simulink model "CAL_3a"  (R2023a)
settings: Solver=ode4  StartTime=0.0  StopTime=105  FixedStep=0.005  RelTol=1e-3
InitFcn:
  | CAL3
values from neighbouring files (symbols this model uses):
  K_scheduled = zeros(length(V_op), 2)    [CAL3.m]    (also in CUB.m; DLC2.m; MUS.m; OHZ.m)
  kappa_track = [zeros(200,1); ones(length(theta_circ)-1, 1)/R_track]    [CAL3.m]    (also in DLC2.m = movmean(kappa_raw, 50); MUS.m = [0; 0]; OHZ.m = [0; 0]; RMP.m = [0; 0])
  psi_track = [zeros(200,1); theta_circ(2:end) + pi/2]    [CAL3.m]    (also in MUS.m = [0; 0]; OHZ.m = [0; 0]; RMP.m = [0; 0]; SLA.m = atan2(dy_ds, dx_ds))
  s_track = [0; cumsum(sqrt(dx.^2 + dy.^2))]    [CAL3.m]    (also in MUS.m = [0; 2000]; OHZ.m = [0; 2000]; RMP.m = [0; 2000]; SLA.m)
  V_op = 5:5:85    [CAL3.m]    (also in CUB.m; DLC2.m; MUS.m; OHZ.m)
  V_profile = conv(V_profile, ones(window_size,1)/window_size, 'same')    [CAL3.m]    (also in SLA.m = u_ms * ones(size(s_track)))
  X_track = [linspace(0, runway_length, 200)'; runway_length + R_track * cos(theta_circ(2:end))]    [CAL3.m]    (also in CUB.m = [0; 5000]; DLC2.m = 0:0.1:total_track_length; MUS.m = [0; 2000]; OHZ.m = [0; 2000])
  Y_track = [zeros(200, 1); R_track + R_track * sin(theta_circ(2:end))]    [CAL3.m]    (also in CUB.m = [0; 0]; DLC2.m = zeros(size(X_track)); MUS.m = [0; 0]; OHZ.m = [0; 0])
undefined symbols (not defined in the file or in its folder): veh_params
libraries: simulink x2, slpidlib x1
(part 2 of 2)

== matlab function CAL_3a/Scopes/MATLAB Function1 ==
  settings: updateMethod=DISCRETE
  data: delta input; psi input; psi_ref input; Fx input; Fy input; Fz input; Trl input; Trr input; Tf_f input; Trl_f input; Trr_f input; w_vec input; vx input; vy input; ax input; ay input
function vehicle_frame_plotter(delta, psi, psi_ref, Fx, Fy, Fz, Trl, Trr, Tf_f, Trl_f, Trr_f, w_vec, vx, vy, ax, ay)
    coder.extrinsic('figure', 'plot', 'hold', 'axis', 'title', 'set', 'drawnow', 'patch', 'text', 'line', 'quiver', 'sprintf');
    
    persistent hWheels hSteer hSpokes hPsiRef hPsiAct hFlags hTqFlags hMotors hAxleFront hCircles hGdots hSwLabel hRwLabel hAngleLabel hVelArrow hAccArrow hVelText hAccText hCrosshairs counter
    
    if isempty(counter)
        % =====================================================================
        % STRICT CODER INITIALIZATION
        % =====================================================================
        counter = 0;
        hSteer = 0.0; hPsiRef = 0.0; hPsiAct = 0.0; hAxleFront = 0.0;
        hWheels = zeros(1,4); hFlags = zeros(1,4); hTqFlags = zeros(1,2); hMotors = zeros(1,2);
        hSpokes = zeros(1,3); hCircles = zeros(1,4); hGdots = zeros(1,4);
        hSwLabel = 0.0; hRwLabel = 0.0; hAngleLabel = 0.0;
        hVelArrow = 0.0; hAccArrow = 0.0; hVelText = 0.0; hAccText = 0.0;
        hCrosshairs = zeros(1,2);
        
        figure('Name', 'Vehicle Frame Telemetry - Car A', 'Color', 'w', 'Position', [100, 100, 750, 750]);
        hold on;
        
        % Chassis Outline & Front Axle
        plot([-1, 1, 1, -1, -1], [2, 2, -2, -2, 2], 'k', 'LineWidth', 2);
        hAxleFront = double(line([1, -1], [1.5, 1.5], 'Color', [0.2 0.2 0.2], 'LineWidth', 2));
        
        % Wheels Array Setup [FL, FR, RL, RR]
        for i = 1:4; hWheels(i) = double(patch(0, 0, [0.3 0.3 0.3])); end
        
        % =====================================================================
        % FRICTION CIRCLES, STEERING WHEEL, & YAW VECTORS
        % =====================================================================
        th_c = 0:0.1:2*pi;
        circle_x = cos(th_c); circle_y = sin(th_c);
        c_pos = [-2.0, 2.3; 2.0, 2.3; -2.0, -2.3; 2.0, -2.3]; 
        for i = 1:4
            hCircles(i) = double(plot(c_pos(i,1) + 0.5*circle_x, c_pos(i,2) + 0.5*circle_y, 'Color', [0.6 0 0.6], 'LineStyle', '--', 'LineWidth', 1.2));
            hGdots(i) = double(plot(c_pos(i,1), c_pos(i,2), 'mo', 'MarkerFaceColor', 'm', 'MarkerSize', 5));
        end
        
        hSteer = double(plot(0.4*cos(th_c), 0.4*sin(th_c) + 0.5, 'k', 'LineWidth', 3));
        hSpokes(1) = double(line([0, 0], [0.5, 0.5], 'Color', 'k', 'LineWidth', 2.5));
        hSpokes(2) = double(line([0, 0], [0.5, 0.5], 'Color', 'k', 'LineWidth', 2.5));
        hSpokes(3) = double(line([0, 0], [0.5, 0.5], 'Color', 'k', 'LineWidth', 2.5));
        
        hPsiRef = double(quiver(0, 1.8, 0, 0.8, 'r', 'LineWidth', 2.5, 'MaxHeadSize', 2));
        hPsiAct = double(quiver(0, 1.8, 0, 0.8, 'b', 'LineWidth', 2.5, 'MaxHeadSize', 2));
        
        for i = 1:4; hFlags(i) = double(text(0, 0, '', 'FontSize', 8, 'BackgroundColor', [1 1 1 0.8], 'EdgeColor', 'k')); end
        
        % =====================================================================
        % VEHICLE A POWERTRAIN GRAPHIC (Dual Motors)
        % =====================================================================
        m_b = [-.15, .15, .15, -.15]; m_w = [.2, .2, -.2, -.2];
        hMotors(1) = double(patch(m_b - 0.6, m_w - 1.5, [0.5 0.5 0.5])); % Left Motor
        hMotors(2) = double(patch(m_b + 0.6, m_w - 1.5, [0.5 0.5 0.5])); % Right Motor
        
        hTqFlags(1) = double(text(-0.6, -0.9, '', 'FontSize', 10, 'FontWeight', 'bold', 'HorizontalAlignment', 'center'));
        hTqFlags(2) = double(text(0.6, -0.9, '', 'FontSize', 10, 'FontWeight', 'bold', 'HorizontalAlignment', 'center'));
        
        % Labels
        hSwLabel = double(text(0, 1.2, '', 'FontSize', 9, 'FontWeight', 'bold', 'HorizontalAlignment', 'center'));
        hRwLabel = double(text(0, 1.65, '', 'FontSize', 9, 'FontWeight', 'bold', 'HorizontalAlignment', 'center', 'Color', [0 0.5 0]));
        hAngleLabel = double(text(0, 2.8, '', 'FontSize', 10, 'FontWeight', 'bold', 'HorizontalAlignment', 'center', 'Color', [0.4 0 0.6]));

        % =====================================================================
        % SHARED-ORIGIN VELOCITY & ACCELERATION VECTORS
        % =====================================================================
        hCrosshairs(1) = double(plot([-2.0 2.0], [-3.8 -3.8], 'k:', 'Color', [0.7 0.7 0.7]));
        hCrosshairs(2) = double(plot([0 0], [-4.2 -1.8], 'k:', 'Color', [0.7 0.7 0.7]));

        hVelArrow = double(quiver(0, -3.8, 0, 0, 'Color', [0 0.4 0.8], 'LineWidth', 2.5, 'MaxHeadSize', 2, 'AutoScale', 'off'));
        hAccArrow = double(quiver(0, -3.8, 0, 0, 'Color', [0.8 0.3 0], 'LineWidth', 2.5, 'MaxHeadSize', 2, 'AutoScale', 'off'));

        hVelText = double(text(-2.0, -4.3, '', 'FontSize', 9, 'FontWeight', 'bold', 'HorizontalAlignment', 'center', 'Color', [0 0.4 0.8]));
        hAccText = double(text(2.0, -4.3, '', 'FontSize', 9, 'FontWeight', 'bold', 'HorizontalAlignment', 'center', 'Color', [0.8 0.3 0]));
        
        axis([-4.5 4.5 -4.5 4.5]); axis equal; grid on;
        title('Dynamics - Car A (Dual Motor): Forces & Friction Circles');
    end
    counter = counter + 1;
    
    % --- UPDATE LOOP ---
    if mod(counter, 10) == 0
        R_delta = [cos(delta) -sin(delta); sin(delta) cos(delta)];
        w_orig = [-.2 .2 .2 -.2; .4 .4 -.4 -.4]; 
        w_rot = R_delta * w_orig;
        
        set(hWheels(1), 'XData', w_rot(1,:) - 1, 'YData', w_rot(2,:) + 1.5); 
        set(hWheels(2), 'XData', w_rot(1,:) + 1, 'YData', w_rot(2,:) + 1.5); 
        set(hWheels(3), 'XData', w_orig(1,:) - 1, 'YData', w_orig(2,:) - 1.5); 
        set(hWheels(4), 'XData', w_orig(1,:) + 1, 'YData', w_orig(2,:) - 1.5); 
        
        set(hAxleFront, 'XData', [mean(w_rot(1,:) - 1), mean(w_rot(1,:) + 1)], 'YData', [mean(w_rot(2,:) + 1.5), mean(w_rot(2,:) + 1.5)]);
        
        sw_a = delta * 14; 
        th_sw = (0:0.1:2*pi) + sw_a;
        set(hSteer, 'XData', 0.4*cos(th_sw), 'YData', 0.4*sin(th_sw) + 0.5);
        spk = [0, pi, 1.5*pi] + sw_a;
        for j=1:3; set(hSpokes(j), 'XData', [0, 0.4*cos(spk(j))], 'YData', [0.5, 0.5 + 0.4*sin(spk(j))]); end
        
        set(hSwLabel, 'String', sprintf('SW: %.1f deg', sw_a * 180/pi));
        set(hRwLabel, 'String', sprintf('RW: %.1f deg', delta * 180/pi));
        
        psi_e = psi_ref - psi; 
        set(hPsiRef, 'UData', 0.8*sin(psi_e), 'VData', 0.8*cos(psi_e));
        set(hPsiAct, 'UData', 0, 'VData', 0.8);
        set(hAngleLabel, 'String', sprintf('Sideslip: %.1f deg', psi_e * 180/pi));
        
        fb = [abs(Tf_f/2), abs(Tf_f/2), abs(Trl_f), abs(Trr_f)]; 
        mu = 1.0;
        c_pos = [-2.0, 2.3; 2.0, 2.3; -2.0, -2.3; 2.0, -2.3]; 
        th_c = 0:0.1:2*pi;
        rpm_vec = w_vec * (30 / pi);
        
        for i = 1:4
            if fb(i) > 5; set(hWheels(i), 'FaceColor', [0.8 0 0]); else set(hWheels(i), 'FaceColor', [0.3 0.3 0.3]); end
            F_max = max(100, mu * Fz(i));
            scale = 0.5 / 6000; 
            set(hCircles(i), 'XData', c_pos(i,1) + F_max*scale*cos(th_c), 'YData', c_pos(i,2) + F_max*scale*sin(th_c));
            set(hGdots(i), 'XData', c_pos(i,1) + Fy(i)*scale, 'YData', c_pos(i,2) + Fx(i)*scale);
        end
        
        % Dual Motor Visualization Logic
        mt = [Trl, Trr]; 
        for k = 1:2
            if mt(k) > 0.1; set(hMotors(k), 'FaceColor', [0 0.7 0]); 
            elseif mt(k) < -0.1; set(hMotors(k), 'FaceColor', [0.7 0 0]); 
            else set(hMotors(k), 'FaceColor', [0.5 0.5 0.5]); end
            
            set(hTqFlags(k), 'String', sprintf('%.1f Nm', mt(k)));
        end
        
        pos = [-4.1, 1.5; 2.8, 1.5; -4.1, -1.5; 2.8, -1.5]; 
        for i = 1:4
            f_str = sprintf('Fx: %.0f\nFy: %.0f\nFz: %.0f\nFric: %.1f\nRPM: %.0f', Fx(i), Fy(i), Fz(i), fb(i), rpm_vec(i));
            set(hFlags(i), 'Position', [pos(i,1), pos(i,2)], 'String', f_str);
        end

        % =====================================================================
        % UPDATE DYNAMIC VECTORS
        % =====================================================================
        vx_kmh = vx * 3.6;
        vy_kmh = vy * 3.6;
        ax_g = ax / 9.81;
        ay_g = ay / 9.81;

        vel_scale = 0.015; 
        acc_scale = 0.8;   

        set(hVelArrow, 'UData', -vy_kmh * vel_scale, 'VData', vx_kmh * vel_scale);
        set(hAccArrow, 'UData', -ay_g * acc_scale, 'VData', ax_g * acc_scale);

        set(hVelText, 'String', sprintf('Vx: %.1f | Vy: %.1f\n[km/h]', vx_kmh, vy_kmh));
        set(hAccText, 'String', sprintf('Ax: %.2f | Ay: %.2f\n[G]', ax_g, ay_g));
        
        drawnow limitrate;
    end
end

== matlab function CAL_3a/Vehicle & Powertrain Plant1/MATLAB Function ==
  data: delta input; Trr_m input; Trl_m input; Trr_f input; Trl_f input; Tf_f input; vx input; vy input; r input; psi input; SOC input; T_batt input; T_motor input; w_fl input; w_fr input; w_rl input; w_rr input; vx_dot output; vy_dot output; r_dot output; X_dot output; Y_dot output; psi_dot output; s_dot output; SOC_dot output; T_batt_dot output; T_mot_dot output; Fz_f_tot output; Fz_r_tot output; Fz_rl output; Fz_rr output; Fx_vec output; Fy_vec output; Fz_vec output; w_vec output; w_dot_vec output; veh_params parameter; I_batt output; Pwr_Elec output
function [vx_dot, vy_dot, r_dot, X_dot, Y_dot, psi_dot, s_dot, SOC_dot, T_batt_dot, T_mot_dot, Fz_f_tot, Fz_r_tot, Fz_rl, Fz_rr, Fx_vec, Fy_vec, Fz_vec, w_vec, w_dot_vec, I_batt, Pwr_Elec] = vehicle_physics_engine(delta, Trr_m, Trl_m, Trr_f, Trl_f, Tf_f, vx, vy, r, psi, SOC, T_batt, T_motor, w_fl, w_fr, w_rl, w_rr, veh_params)
    
    % =========================================================================
    % 0. EXPLICIT OUTPUT INITIALIZATION & SCALAR COERCION 
    % =========================================================================
    vx_dot = 0.0; vy_dot = 0.0; r_dot = 0.0; 
    X_dot = 0.0; Y_dot = 0.0; psi_dot = 0.0; s_dot = 0.0;
    SOC_dot = 0.0; T_batt_dot = 0.0; T_mot_dot = 0.0;
    Fz_f_tot = 0.0; Fz_r_tot = 0.0; Fz_rl = 0.0; Fz_rr = 0.0;
    Fx_vec = zeros(1,4); Fy_vec = zeros(1,4); Fz_vec = zeros(1,4);
    w_vec = zeros(1,4); w_dot_vec = zeros(1,4);
    I_batt = 0.0; 
    Pwr_Elec = 0.0; % NEW: Output initialization for Electrical Power

    % Force scalar inputs (strips undefined array dimensions from Simulink lines)
    delta = delta(1); vx = vx(1); vy = vy(1); r = r(1); psi = psi(1);
    Trr_m = Trr_m(1); Trl_m = Trl_m(1); Trr_f = Trr_f(1); Trl_f = Trl_f(1); Tf_f = Tf_f(1);
    SOC = SOC(1); T_batt = T_batt(1); T_motor = T_motor(1);
    w_fl = w_fl(1); w_fr = w_fr(1); w_rl = w_rl(1); w_rr = w_rr(1);

    % =========================================================================
    % HIGH-FIDELITY EV VEHICLE DYNAMICS PLANT MODEL
    % =========================================================================
    
    % ---------------------------------------------------------------------
    % 1. UNPACK CENTRALIZED PARAMETERS
    % ---------------------------------------------------------------------
    m = veh_params.m(1); Iz = veh_params.Iz(1); lf = veh_params.lf(1); lr = veh_params.lr(1); L = veh_params.L(1);
    tw = veh_params.tw(1); h_cg = veh_params.h_cg(1); Rw = veh_params.Rw(1); Iw = veh_params.Iw(1); 
    G = veh_params.G(1); g = veh_params.g(1); rho = veh_params.rho(1); CdA = veh_params.CdA(1);
    roll_bias_f = veh_params.roll_bias_f(1); 
    
    mu_max = veh_params.mu_max(1); C_rr = veh_params.C_rr(1);
    ks_f = veh_params.ks_f(1)/2; ks_r = veh_params.ks_r(1)/2;
    C_tire = veh_params.C_tire(1); E_tire = veh_params.E_tire(1);
    
    if abs(vx) < 0.5
        vx_safe = 0.5 * sign(vx + 1e-6); 
    else
        vx_safe = vx;
    end
    
    F_aero_drag = 0.5 * rho * CdA * vx_safe * abs(vx_safe);
    
    % ---------------------------------------------------------------------
    % 2. DYNAMIC TIRE PEAK CALIBRATION
    % ---------------------------------------------------------------------
    Fz_axle_f_static = m * g * (lr / L); 
    Fz_axle_r_static = m * g * (lf / L); 
    
    D_tire_f = mu_max * (Fz_axle_f_static / 2); 
    D_tire_r = mu_max * (Fz_axle_r_static / 2); 
    
    B_tire_f = ks_f / (C_tire * D_tire_f * 2); 
    B_tire_r = ks_r / (C_tire * D_tire_r * 2); 
    
    % ---------------------------------------------------------------------
    % 3. 3D WEIGHT TRANSFER 
    % ---------------------------------------------------------------------
    Trr_tot = Trr_m * G + Trr_f;
    Trl_tot = Trl_m * G + Trl_f;
    Tf_tot_half = Tf_f / 2; 
    
    Fx_fl_tq = Tf_tot_half / Rw; Fx_fr_tq = Tf_tot_half / Rw;
    Fx_rl_tq = Trl_tot / Rw; Fx_rr_tq = Trr_tot / Rw;
    
    ax_est = ((Fx_fl_tq + Fx_fr_tq + Fx_rl_tq + Fx_rr_tq) - F_aero_drag) / m;
    ay_est = vx_safe * r;
    
    Fz_f_tot = m * g * (lr / L) - m * ax_est * (h_cg / L);
    Fz_r_tot = m * g * (lf / L) + m * ax_est * (h_cg / L);
    
    dFz_y_f = m * ay_est * (h_cg / tw) * roll_bias_f;
    dFz_y_r = m * ay_est * (h_cg / tw) * (1 - roll_bias_f);
    
    Fz_max_f = Fz_axle_f_static * 2.5; 
    Fz_max_r = Fz_axle_r_static * 2.5;
    
    Fz_fl = max(100, min(Fz_max_f, Fz_f_tot / 2 - dFz_y_f));
    Fz_fr = max(100, min(Fz_max_f, Fz_f_tot / 2 + dFz_y_f));
    Fz_rl = max(100, min(Fz_max_r, Fz_r_tot / 2 - dFz_y_r));
    Fz_rr = max(100, min(Fz_max_r, Fz_r_tot / 2 + dFz_y_r));
    Fz_vec = [Fz_fl, Fz_fr, Fz_rl, Fz_rr];
    
    % ---------------------------------------------------------------------
    % 4. VECTOR-SUM PACEJKA COMBINED SLIP MODEL
    % ---------------------------------------------------------------------
    v_hub_fl = vx_safe - (tw / 2) * r; v_hub_fr = vx_safe + (tw / 2) * r;
    v_hub_rl = vx_safe - (tw / 2) * r; v_hub_rr = vx_safe + (tw / 2) * r;
    
    k_fl = (w_fl * Rw - v_hub_fl) / max(abs(v_hub_fl), 1.0);
    k_fr = (w_fr * Rw - v_hub_fr) / max(abs(v_hub_fr), 1.0);
    k_rl = (w_rl * Rw - v_hub_rl) / max(abs(v_hub_rl), 1.0);
    k_rr = (w_rr * Rw - v_hub_rr) / max(abs(v_hub_rr), 1.0);
    
    alpha_fl = delta - atan((vy + lf * r) / max(abs(v_hub_fl), 1.0));
    alpha_fr = delta - atan((vy + lf * r) / max(abs(v_hub_fr), 1.0));
    alpha_rl = -atan((vy - lr * r) / max(abs(v_hub_rl), 1.0));
    alpha_rr = -atan((vy - lr * r) / max(abs(v_hub_rr), 1.0));
    
    sigma_fl = sqrt(k_fl^2 + tan(alpha_fl)^2) + 1e-6;
    sigma_fr = sqrt(k_fr^2 + tan(alpha_fr)^2) + 1e-6;
    sigma_rl = sqrt(k_rl^2 + tan(alpha_rl)^2) + 1e-6;
    sigma_rr = sqrt(k_rr^2 + tan(alpha_rr)^2) + 1e-6;
    
    F_tot_fl = mu_max * Fz_fl * sin(C_tire * atan(B_tire_f * sigma_fl - E_tire * (B_tire_f * sigma_fl - atan(B_tire_f * sigma_fl))));
    F_tot_fr = mu_max * Fz_fr * sin(C_tire * atan(B_tire_f * sigma_fr - E_tire * (B_tire_f * sigma_fr - atan(B_tire_f * sigma_fr))));
    F_tot_rl = mu_max * Fz_rl * sin(C_tire * atan(B_tire_r * sigma_rl - E_tire * (B_tire_r * sigma_rl - atan(B_tire_r * sigma_rl))));
    F_tot_rr = mu_max * Fz_rr * sin(C_tire * atan(B_tire_r * sigma_rr - E_tire * (B_tire_r * sigma_rr - atan(B_tire_r * sigma_rr))));
    
    Fx_fl = F_tot_fl * (k_fl / sigma_fl) - C_rr * Fz_fl * tanh(v_hub_fl * 10);
    Fx_fr = F_tot_fr * (k_fr / sigma_fr) - C_rr * Fz_fr * tanh(v_hub_fr * 10);
    Fx_rl = F_tot_rl * (k_rl / sigma_rl) - C_rr * Fz_rl * tanh(v_hub_rl * 10);
    Fx_rr = F_tot_rr * (k_rr / sigma_rr) - C_rr * Fz_rr * tanh(v_hub_rr * 10);
    Fx_vec = [Fx_fl, Fx_fr, Fx_rl, Fx_rr];
    
    Fy_fl = F_tot_fl * (tan(alpha_fl) / sigma_fl);
    Fy_fr = F_tot_fr * (tan(alpha_fr) / sigma_fr);
    Fy_rl = F_tot_rl * (tan(alpha_rl) / sigma_rl);
    Fy_rr = F_tot_rr * (tan(alpha_rr) / sigma_rr);
    Fy_vec = [Fy_fl, Fy_fr, Fy_rl, Fy_rr];
    
    % ---------------------------------------------------------------------
    % 5. CHASSIS & WHEEL INTEGRATORS
    % ---------------------------------------------------------------------
    w_fl_dot = (-abs(Tf_f / 2) * sign(w_fl) - Fx_fl * Rw) / Iw;
    w_fr_dot = (-abs(Tf_f / 2) * sign(w_fr) - Fx_fr * Rw) / Iw;
    w_rl_dot = (Trl_m * G - abs(Trl_f) * sign(w_rl) - Fx_rl * Rw) / Iw;
    w_rr_dot = (Trr_m * G - abs(Trr_f) * sign(w_rr) - Fx_rr * Rw) / Iw;
    w_dot_vec = [w_fl_dot, w_fr_dot, w_rl_dot, w_rr_dot];
    w_vec = [w_fl, w_fr, w_rl, w_rr];
    
    sum_Fx = (Fx_fl + Fx_fr) * cos(delta) - (Fy_fl + Fy_fr) * sin(delta) + Fx_rl + Fx_rr;
    vx_dot = (sum_Fx - F_aero_drag) / m + vy * r;
    
    sum_Fy = (Fy_fl + Fy_fr) * cos(delta) + (Fx_fl + Fx_fr) * sin(delta) + Fy_rl + Fy_rr;
    vy_dot = sum_Fy / m - vx_safe * r;
    
    M_front = lf * ((Fy_fl + Fy_fr) * cos(delta) + (Fx_fl + Fx_fr) * sin(delta));
    M_rear  = -lr * (Fy_rl + Fy_rr);
    M_tv    = (Fx_rr - Fx_rl) * (tw / 2); 
    r_dot  = (M_front + M_rear + M_tv) / Iz;
    
    X_dot   = vx_safe * cos(psi) - vy * sin(psi);
    Y_dot   = vx_safe * sin(psi) + vy * cos(psi);
    psi_dot = r;
    s_dot   = vx_safe;
    
    % ---------------------------------------------------------------------
    % 6. THERMALS & SOC (R-INT BATTERY MODEL)
    % ---------------------------------------------------------------------
    P_mech = (Trr_m + Trl_m) * G * (vx_safe / Rw);
    P_elec = P_mech; 
    
    if P_mech > 500
        P_elec = P_mech / 0.90; 
    elseif P_mech < -500
        P_elec = P_mech * 0.90; 
    end
    
    V_oc = veh_params.V_pack; 
    R_int = 0.015;            
    
    discriminant = V_oc^2 - 4 * R_int * P_elec;
    
    if discriminant < 0
        discriminant = 0;
    end
    
    I_curr = (V_oc - sqrt(discriminant)) / (2 * R_int);
    
    % NEW OUTPUTS
    I_batt = I_curr;
    Pwr_Elec = P_elec;
    
    SOC_dot = -I_curr / (veh_params.Cap_Ah * 3600);
    
    T_batt_dot = ((I_curr^2) * R_int - veh_params.hA_cool_batt * (T_batt - veh_params.T_coolant_batt)) / (veh_params.m_batt * veh_params.cp_batt);
    T_mot_dot  = (abs(P_elec - P_mech) - veh_params.hA_cool_motor * (T_motor - veh_params.T_ambient)) / (veh_params.m_motor * veh_params.cp_motor);
end

== matlab function CAL_3a/Vehicle Control Unit (VCU)/MATLAB Function ==
  settings: updateMethod=DISCRETE
  data: delta_curr input; pedal input; T_rr_motor_raw output; vx_curr input; vy_curr input; r_curr input; kappa_ref input; Fz_f_total input; Fz_r_total input; Fz_rl input; Fz_rr input; SOC input; T_batt input; T_motor input; V_op parameter; K_scheduled parameter; T_rl_motor_raw output; T_rr_fric output; w_vec input; T_rl_fric output; T_f_fric output; Mz_cmd output; r_ref output
function [T_rr_motor_raw, T_rl_motor_raw, T_rr_fric, T_rl_fric, T_f_fric, Mz_cmd, r_ref] = vcu_allocator(delta_curr, pedal, vx_curr, vy_curr, r_curr, kappa_ref, Fz_f_total, Fz_r_total, Fz_rl, Fz_rr, SOC, T_batt, T_motor, V_op, K_scheduled, w_vec)
T_rr_motor_raw = 0.0;
T_rl_motor_raw = 0.0;
T_rr_fric = 0.0;
T_rl_fric = 0.0;
T_f_fric = 0.0;
Mz_cmd = 0.0;

Rw = 0.34; tw = 1.65; G = 10; mu_max = 1.2;

% --- Per-Motor Limits (Total System = 500 kW, 800 Nm) ---
P_motor_base = 250000; % 250 kW per motor
T_motor_max = 400;     % 400 Nm per motor
T_fric_max_per_wheel = 3500;
% --------------------------------------------------------

% --- Battery and Thermal Derating ---
T_batt_cal = [-10, 0, 15, 45, 55, 60]; P_derate_batt_cal = [0, 0.5, 1.0, 1.0, 0.2, 0];
T_motor_cal = [30, 90, 110, 130, 150]; P_derate_motor_cal = [1.0, 1.0, 0.8, 0.2, 0];
SOC_vec = [0, 0.05, 0.15, 0.85, 0.95, 1.0];
P_derate_SOC_dis = [0, 0.1, 1.0, 1.0, 1.0, 1.0]; P_derate_SOC_chg = [1.0, 1.0, 1.0, 1.0, 0.1, 0];

derate_T_batt = interp1(T_batt_cal, P_derate_batt_cal, T_batt(1), 'linear', 0);
derate_T_mot = interp1(T_motor_cal, P_derate_motor_cal, T_motor(1), 'linear', 0);
derate_T_total = min(derate_T_batt, derate_T_mot);

derate_S_dis = interp1(SOC_vec, P_derate_SOC_dis, SOC(1), 'linear', 0);
derate_S_chg = interp1(SOC_vec, P_derate_SOC_chg, SOC(1), 'linear', 0);

P_avail_dis = P_motor_base * min(derate_T_total, derate_S_dis);
P_avail_chg = P_motor_base * min(derate_T_total, derate_S_chg);

vx_lqr = max(vx_curr(1), 5.0);

% --- Speed-based Torque Vectoring Blending (45 km/h to 50 km/h) ---
vx_kmh = vx_curr(1) * 3.6;
tv_blend_lower = 45.0;
tv_blend_upper = 50.0;
if vx_kmh >= tv_blend_upper
    tv_blend = 1.0;
elseif vx_kmh <= tv_blend_lower
    tv_blend = 0.0;
else
    tv_blend = (vx_kmh - tv_blend_lower) / (tv_blend_upper - tv_blend_lower);
end

% --- LQR Yaw Moment Calculation ---
K_dyn_1 = interp1(V_op, K_scheduled(:,1), vx_lqr, 'linear', 'extrap');
K_dyn_2 = interp1(V_op, K_scheduled(:,2), vx_lqr, 'linear', 'extrap');

% =========================================================================
% 1. DYNAMIC ACKERMANN REFERENCE
% =========================================================================
L = 2.6;            % Wheelbase
K_us = 0.0015;      % Small understeer gradient (optional)
r_ref_raw = (vx_lqr * delta_curr(1)) / (L * (1 + K_us * vx_lqr^2));

% =========================================================================
% 2. PHYSICAL YAW RATE BOUNDING (The Jitter Fix)
% =========================================================================
g = 9.81;
% Calculate the absolute maximum yaw rate the tires can sustain
% based on current speed and track friction (r_max = mu * g / Vx)
% We use 0.95 as a safety margin to prevent fighting the TCS limiters.
r_max_phys = (mu_max * g * 0.95) / vx_lqr;

% Clamp the reference so the LQR never demands an impossible turn
r_ref = max(-r_max_phys, min(r_max_phys, r_ref_raw));

% =========================================================================
TV_Bite_Factor = 1;
vy_factor = 1;
Mz_req = tv_blend * -(vy_factor * K_dyn_1(1) * vy_curr(1) + TV_Bite_Factor * K_dyn_2(1) * (r_curr(1) - r_ref));

Mz_cmd = max(-2500, min(2500, Mz_req));
T_delta_wheel_raw = max(-1500, min(1500, (Mz_cmd * Rw) / tw));

% =========================================================================
% --- DYNAMIC MOTOR POWER LIMITS (Hyperbolic Torque Derating) ---
% =========================================================================
% Calculate actual motor speed from wheel speed (rad/s)
% w_vec = [w_fl, w_fr, w_rl, w_rr]
w_motor_rl = max(abs(w_vec(3) * G), 0.1); % Prevent div-by-zero at standstill
w_motor_rr = max(abs(w_vec(4) * G), 0.1);

% Power-limited torque curve: T_max = P_max / w
T_limit_rl_dis = P_avail_dis / w_motor_rl;
T_limit_rr_dis = P_avail_dis / w_motor_rr;
T_limit_rl_chg = P_avail_chg / w_motor_rl;
T_limit_rr_chg = P_avail_chg / w_motor_rr;

% Final motor bounds (Minimum of Inverter current limit and Power limit)
T_motor_lim_rl_dis = min(T_motor_max, T_limit_rl_dis);
T_motor_lim_rr_dis = min(T_motor_max, T_limit_rr_dis);
T_motor_lim_rl_chg = max(-T_motor_max, -T_limit_rl_chg);
T_motor_lim_rr_chg = max(-T_motor_max, -T_limit_rr_chg);

% =========================================================================
T_grip_lim_rl_wheel = mu_max * Fz_rl(1) * Rw * 0.90;
T_grip_lim_rr_wheel = mu_max * Fz_rr(1) * Rw * 0.90;

% Combine physical motor limits with dynamic grip limits
T_max_rl_motor = min(T_motor_lim_rl_dis, T_grip_lim_rl_wheel / G);
T_max_rr_motor = min(T_motor_lim_rr_dis, T_grip_lim_rr_wheel / G);
T_min_rl_motor = max(T_motor_lim_rl_chg, -T_grip_lim_rl_wheel / G);
T_min_rr_motor = max(T_motor_lim_rr_chg, -T_grip_lim_rr_wheel / G);

weight_rl = Fz_rl(1) / max(1, (Fz_rl(1) + Fz_rr(1)));
weight_rr = Fz_rr(1) / max(1, (Fz_rl(1) + Fz_rr(1)));

% --- DRIVE MODE ---
if pedal(1) >= 0
    % Total requested drive torque, limited by combined max capabilities
    T_req_total_motor = pedal(1) * (T_max_rl_motor + T_max_rr_motor);
    T_rr_base_motor = T_req_total_motor * weight_rr;
    T_rl_base_motor = T_req_total_motor * weight_rl;
    
    T_rr_ideal = max(T_min_rr_motor, min(T_max_rr_motor, T_rr_base_motor + (T_delta_wheel_raw/G)));
    T_rl_ideal = max(T_min_rl_motor, min(T_max_rl_motor, T_rl_base_motor - (T_delta_wheel_raw/G)));
    
    % Traction Control (TCS) - Virtual Differential Logic Update
    v_hub_rl = max(vx_curr(1) - (tw/2)*r_curr(1), 1.0);
    v_hub_rr = max(vx_curr(1) + (tw/2)*r_curr(1), 1.0);
    
    kappa_rl = (w_vec(3)*Rw - v_hub_rl) / v_hub_rl;
    kappa_rr = (w_vec(4)*Rw - v_hub_rr) / v_hub_rr;
    
    slip_target = 0.10;
    Kp_tcs = 1000;
    
    % NEW LOGIC: Find the worst-case slip across the axle
    worst_kappa_rear = max(kappa_rl, kappa_rr);
    
    if worst_kappa_rear > slip_target
        % Calculate a single, unified torque penalty
        T_tcs_penalty = Kp_tcs * (worst_kappa_rear - slip_target);
        
        % Apply the EXACT same penalty to BOTH motors. 
        % This links them together and kills asymmetric thrust during a single-wheel slip.
        T_rl_ideal = max(0, T_rl_ideal - T_tcs_penalty);
        T_rr_ideal = max(0, T_rr_ideal - T_tcs_penalty);
    end
    
    T_rr_fric = 0; T_rl_fric = 0; T_f_fric = 0;

% --- BRAKE MODE ---
else
    bias_f = 0.70;
    total_grip_cap_wheel = mu_max * (Fz_f_total(1) + Fz_r_total(1)) * Rw * 0.90;
    
    T_req_total_wheel = pedal(1) * total_grip_cap_wheel;
    T_req_front_wheel = T_req_total_wheel * bias_f;
    T_req_rear_wheel  = T_req_total_wheel * (1 - bias_f);
    
    T_f_fric = max(-mu_max * Fz_f_total(1) * Rw * 0.90, T_req_front_wheel);
    
    T_base_rr = max(-(T_grip_lim_rr_wheel - abs(T_delta_wheel_raw)), T_req_rear_wheel * weight_rr);
    T_base_rl = max(-(T_grip_lim_rl_wheel - abs(T_delta_wheel_raw)), T_req_rear_wheel * weight_rl);
    
    T_rr_ideal_wheel = T_base_rr + T_delta_wheel_raw;
    T_rl_ideal_wheel = T_base_rl - T_delta_wheel_raw;
    
    % Anti-Lock Braking (ABS)
    v_hub_fl = max(vx_curr(1) - (tw/2)*r_curr(1), 1.0);
    v_hub_fr = max(vx_curr(1) + (tw/2)*r_curr(1), 1.0);
    v_hub_rl = max(vx_curr(1) - (tw/2)*r_curr(1), 1.0);
    v_hub_rr = max(vx_curr(1) + (tw/2)*r_curr(1), 1.0);
    
    kappa_fl = (w_vec(1)*Rw - v_hub_fl) / v_hub_fl;
    kappa_fr = (w_vec(2)*Rw - v_hub_fr) / v_hub_fr;
    kappa_rl = (w_vec(3)*Rw - v_hub_rl) / v_hub_rl;
    kappa_rr = (w_vec(4)*Rw - v_hub_rr) / v_hub_rr;
    
    slip_limit_abs = -0.10;
    Kp_abs = 5000;
    
    worst_kappa_f = min(kappa_fl, kappa_fr);
    if worst_kappa_f < slip_limit_abs
        T_f_fric = min(0, T_f_fric - Kp_abs * (worst_kappa_f - slip_limit_abs));
    end
    
    if kappa_rl < slip_limit_abs
        T_rl_ideal_wheel = min(0, T_rl_ideal_wheel - Kp_abs * (kappa_rl - slip_limit_abs));
    end
    if kappa_rr < slip_limit_abs
        T_rr_ideal_wheel = min(0, T_rr_ideal_wheel - Kp_abs * (kappa_rr - slip_limit_abs));
    end
    
    T_rr_ideal = max(T_min_rr_motor, min(T_max_rr_motor, T_rr_ideal_wheel / G));
    T_rl_ideal = max(T_min_rl_motor, min(T_max_rl_motor, T_rl_ideal_wheel / G));
    
    T_rr_fric = max(-T_fric_max_per_wheel, min(0, T_rr_ideal_wheel - (T_rr_ideal * G)));
    T_rl_fric = max(-T_fric_max_per_wheel, min(0, T_rl_ideal_wheel - (T_rl_ideal * G)));
    
    if vx_curr(1) < 2.0
        T_f_fric = 0; T_rr_fric = 0; T_rl_fric = 0;
        T_rr_ideal = 0; T_rl_ideal = 0;
    end
end

T_rr_motor_raw = T_rr_ideal;
T_rl_motor_raw = T_rl_ideal;

end

== matlab function CAL_3a/Track & Environment references/MATLAB Function ==
  settings: updateMethod=DISCRETE
  data: X_curr input; v_ref output; Y_curr input; psi_curr input; vx_curr input; kappa_ref output; psi_ref output; delta_cmd output; X_track parameter; Y_track parameter; s_track parameter; V_profile parameter; kappa_track parameter; psi_track parameter; sim_time input; Fz_vec input; veh_params parameter; recovery_active output
function [v_ref, kappa_ref, psi_ref, delta_cmd, recovery_active] = pure_pursuit_planner(X_curr, Y_curr, psi_curr, vx_curr, X_track, Y_track, s_track, V_profile, kappa_track, psi_track, sim_time, Fz_vec, veh_params)
    
    persistent recovery_start_time tube_exceeded prev_idx delta_cmd_prev
    if isempty(recovery_start_time); recovery_start_time = -10; end
    if isempty(tube_exceeded); tube_exceeded = 0; end
    if isempty(prev_idx); prev_idx = 1; end
    if isempty(delta_cmd_prev); delta_cmd_prev = 0.0; end
    
    % --- 1. FIND NEAREST POINT ON SPATIAL TRACK (LOCAL SEARCH) ---
    search_window_end = min(length(X_track), prev_idx + 200);
    dist_sq = (X_track(prev_idx:search_window_end) - X_curr).^2 + ...
              (Y_track(prev_idx:search_window_end) - Y_curr).^2;
    [min_dist_sq, local_min_idx] = min(dist_sq);
    min_idx = prev_idx + local_min_idx - 1;
    prev_idx = min_idx;
    e_ct = sqrt(min_dist_sq); 
    
    % --- 2. RELAXED TUBE LOGIC FOR ISO 4138 ---
    tube_limit = 500.0; 
    if e_ct > tube_limit && tube_exceeded == 0
        tube_exceeded = 1;
        recovery_start_time = sim_time;
    end
    if sim_time - recovery_start_time < 1.0 && tube_exceeded == 1
        recovery_active = 1; v_ref = 0.0; delta_cmd = 0.0; kappa_ref = 0.0; psi_ref = psi_track(min_idx);
        return; 
    else
        recovery_active = 0;
        if e_ct < 2.0; tube_exceeded = 0; end 
    end
    
    % --- 3. PURE PURSUIT LOGIC ---
    vx_safe = max(vx_curr, 2.0); 
    Ld = max(12.0, 1.0 * vx_safe); 
    
    idx_target = min_idx;
    while idx_target < length(s_track) && (s_track(idx_target) - s_track(min_idx)) < Ld
        idx_target = idx_target + 1;
    end
    
    X_target = X_track(idx_target); 
    Y_target = Y_track(idx_target);
    
    alpha = atan2(Y_target - Y_curr, X_target - X_curr) - psi_curr;
    alpha = mod(alpha + pi, 2*pi) - pi;
    
    % Raw geometric request
    delta_raw = atan2(2 * veh_params.L * sin(alpha), Ld);
    
    % =====================================================================
    % --- 4. REALISTIC TEST DRIVER BEHAVIOR (ANTI-YANK) ---
    % =====================================================================
    dt = 0.001; % Assuming 1ms Simulink solver step
    
    % A. Human Steering Rate Limiter
    % Restricts the virtual driver from turning the wheel faster than 15 deg/sec.
    % This stops the violent yanking when tracking error grows.
    max_rate_rad_sec = 15.0 * (pi / 180); 
    delta_rate = (delta_raw - delta_cmd_prev) / dt;
    delta_rate_clamped = max(-max_rate_rad_sec, min(max_rate_rad_sec, delta_rate));
    delta_smoothed = delta_cmd_prev + delta_rate_clamped * dt;
    
    % B. Pacejka Saturation Guard (Speed-Dependent Cap)
    % A real driver knows that adding 20+ degrees of steering at 100 km/h 
    % just plows the tires. We cap the maximum absolute steering angle to ~12 degrees
    % to force the driver to "hold the line" and let the car understeer cleanly.
    max_steer_rad = 12.0 * (pi / 180);
    delta_cmd = max(-max_steer_rad, min(max_steer_rad, delta_smoothed));
    
    % Save state for next millisecond
    delta_cmd_prev = delta_cmd;
    % =====================================================================

    % --- 5. CONTINUOUS ACCELERATION TARGET ---
    v_ref = V_profile(min_idx);
    kappa_ref = (2 * sin(alpha)) / Ld;
    psi_ref = psi_track(min_idx);
end
